simulink model "ACC"  (R2022b)
settings: Solver=FixedStepDiscrete  StartTime=0.0  StopTime=10.0  FixedStep=0.01  RelTol=1e-3
libraries: simulink x1
settings Model: DataDictionary=Adaptive_Cruise_Control.sldd  Creator=MAAM  LastModifiedBy=MAAM
settings OptimizationCC: DefaultParameterBehavior=Inlined  UseDivisionForNetSlopeComputation=on  GainParamInheritBuiltInType=on  UseFloatMulNetSlope=on  InlineInvariantSignals=on  PassReuseOutputArgsAs=Individual arguments  ZeroExternalMemoryAtStartup=off  ZeroInternalMemoryAtStartup=off  NoFixptDivByZeroProtection=on  EfficientFloat2IntCast=on  LifeSpan=1  OptimizeBlockOrder=speed  DifferentSizesBufferReuse=on  EfficientTunableParamExpr=on
settings DebuggingCC: ParameterTunabilityLossMsg=error
settings HardwareCC: ProdBitPerPointer=32  ProdBitPerSizeT=32  ProdBitPerPtrDiffT=32  ProdLargestAtomicInteger=Long  ProdLargestAtomicFloat=Double  ProdWordSize=32  ProdLongLongMode=on  ProdHWDeviceType=ARM Compatible->ARM Cortex-M
settings SFSimCC: MATLABDynamicMemAlloc=off
settings RTWCC: Description=Embedded Coder  SystemTargetFile=ert.tlc  GenCodeOnly=on  TemplateMakefile=ert_default_tmf
settings CodeAppCC: ForceParamTrailComments=on  IgnoreCustomStorageClasses=off  OperatorAnnotations=on  SimulinkDataObjDesc=on  SFDataObjDesc=on  CustomSymbolStrGlobalVar=rt$N$M  CustomSymbolStrType=$N$M  CustomSymbolStrFcn=$N$M$F  CustomSymbolStrMacro=$N$M  InsertBlockDesc=on
settings ERTTargetCC: TargetLangStandard=C99 (ISO)  GenerateSampleERTMain=on  IncludeMdlTerminateFcn=off  CombineSignalStateStructs=on  SupportAbsoluteTime=off  SupportComplex=off  SupportNonInlinedSFcns=on  InlinedParameterPlacement=NonHierarchical  ERTCustomFileTemplate=example_file_process.tlc  ERTFilePackagingFormat=CompactWithDataFile

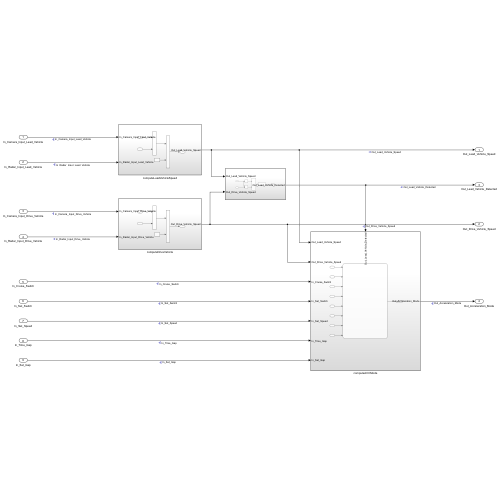
[thumbnail: Simulink's stored preview of the top-level diagram]
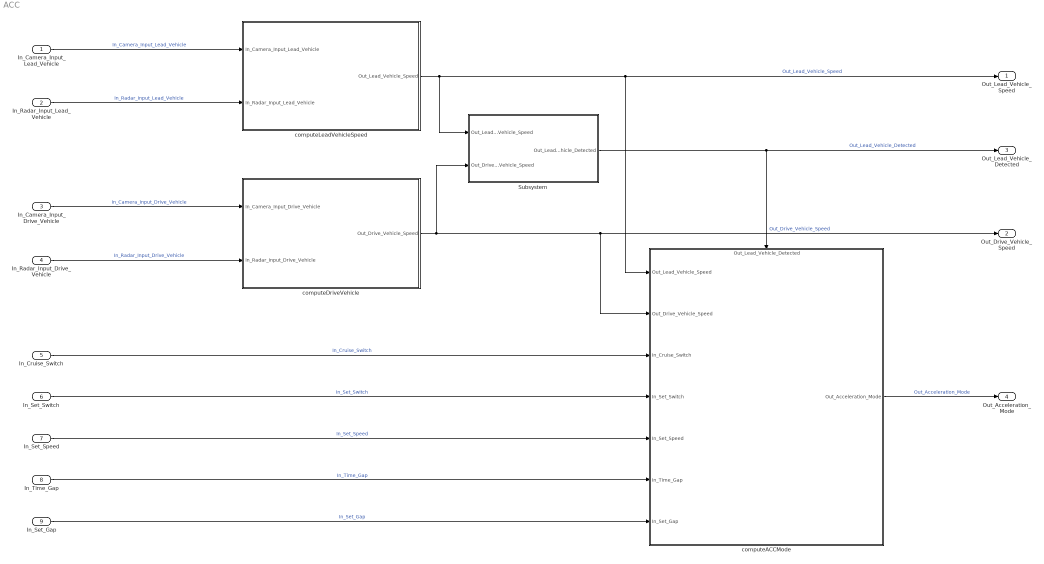
== system ACC ==
  In_Camera_Input_Lead_Vehicle : Inport  OutDataTypeStr=uint8
  In_Radar_Input_Lead_Vehicle : Inport  Port=2  OutDataTypeStr=uint8
  In_Camera_Input_Drive_Vehicle : Inport  Port=3  OutDataTypeStr=uint8
  In_Radar_Input_Drive_Vehicle : Inport  Port=4  OutDataTypeStr=uint8
  In_Cruise_Switch : Inport  Port=5  OutDataTypeStr=boolean
  In_Set_Switch : Inport  Port=6  OutDataTypeStr=boolean
  In_Set_Speed : Inport  Port=7  OutDataTypeStr=uint8
  In_Time_Gap : Inport  Port=8  OutDataTypeStr=uint8
  In_Set_Gap : Inport  Port=9  OutDataTypeStr=uint8
  Subsystem : Subsystem
  computeACCMode : Subsystem
      settings: PortSchema="{\"entries\":[{\"content\":{\"sides\":[{\"content\":{\"connectorIds\":[\"In1\",\"In2\",\"In3\",\"In4\",\"In5\",\"In6\",\"In7\"]},\"type\":\"ConnectorPlacement.EquallySpacedRectSide\",\"uuid\":\"34e4527d-3073-4040-9a65-5b2192b0ac7a\"},{\"content\":{\"connectorIds\":[\"Out1\"],\"side\":\"RIGHT\"},\"type\":\"ConnectorPlacement.EquallySpacedRectSide\",\"uuid\":\"d28eb757-50b9-4815-93ce-88b039d8e03c\"},{\"content\":{\"connectorIds\":[\"In8\"],\"side\":\"TOP\"},\"type\":\"ConnectorPlacement.EquallySpacedRectSide\",\"uuid\":\"9f5a8a03-fc12-423c-b68a-6a82dedc6e29\"}]},\"type\":\"ConnectorPlacement.EquallySpacedConnector\",\"uuid\":\"64ab1c3b-0e5f-41ed-aa52-f96656837c78\"}],\"packageUris\":[\"http://schema.mathworks.com/mf0/Connector/R2020b\"],\"version\":\"1.0\"}"
  computeDriveVehicle : Subsystem
  computeLeadVehicleSpeed : Subsystem
  Out_Lead_Vehicle_Speed : Outport  OutDataTypeStr=uint8
  Out_Drive_Vehicle_Speed : Outport  Port=2  OutDataTypeStr=uint8
  Out_Lead_Vehicle_Detected : Outport  Port=3  OutDataTypeStr=uint8
  Out_Acceleration_Mode : Outport  Port=4  OutDataTypeStr=uint8
  wires:
  computeLeadVehicleSpeed/1(Out_Lead_Vehicle_Speed) -> Subsystem/1(Out_Lead_Vehicle_Speed), Out_Lead_Vehicle_Speed/1, computeACCMode/1(Out_Lead_Vehicle_Speed)  "Out_Lead_Vehicle_Speed"
  In_Camera_Input_Lead_Vehicle/1 -> computeLeadVehicleSpeed/1(In_Camera_Input_Lead_Vehicle)  "In_Camera_Input_Lead_Vehicle"
  In_Radar_Input_Lead_Vehicle/1 -> computeLeadVehicleSpeed/2(In_Radar_Input_Lead_Vehicle)  "In_Radar_Input_Lead_Vehicle"
  computeDriveVehicle/1(Out_Drive_Vehicle_Speed) -> Out_Drive_Vehicle_Speed/1, computeACCMode/2(Out_Drive_Vehicle_Speed), Subsystem/2(Out_Drive_Vehicle_Speed)  "Out_Drive_Vehicle_Speed"
  computeACCMode/1(Out_Acceleration_Mode) -> Out_Acceleration_Mode/1  "Out_Acceleration_Mode"
  In_Cruise_Switch/1 -> computeACCMode/3(In_Cruise_Switch)  "In_Cruise_Switch"
  In_Set_Switch/1 -> computeACCMode/4(In_Set_Switch)  "In_Set_Switch"
  In_Set_Speed/1 -> computeACCMode/5(In_Set_Speed)  "In_Set_Speed"
  In_Time_Gap/1 -> computeACCMode/6(In_Time_Gap)  "In_Time_Gap"
  In_Set_Gap/1 -> computeACCMode/7(In_Set_Gap)  "In_Set_Gap"
  In_Radar_Input_Drive_Vehicle/1 -> computeDriveVehicle/2(In_Radar_Input_Drive_Vehicle)  "In_Radar_Input_Drive_Vehicle"
  In_Camera_Input_Drive_Vehicle/1 -> computeDriveVehicle/1(In_Camera_Input_Drive_Vehicle)  "In_Camera_Input_Drive_Vehicle"
  Subsystem/1(Out_Lead_Vehicle_Detected) -> Out_Lead_Vehicle_Detected/1, computeACCMode/8(Out_Lead_Vehicle_Detected)  "Out_Lead_Vehicle_Detected"

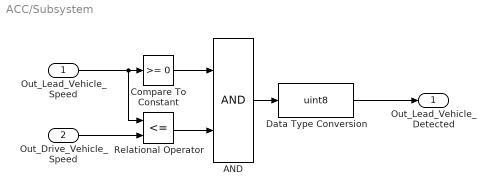
== system ACC/Subsystem ==
  Out_Lead_Vehicle_Speed : Inport  OutDataTypeStr=uint8
  Out_Drive_Vehicle_Speed : Inport  Port=2  OutDataTypeStr=uint8
  AND : Logic  AllPortsSameDT=off  OutDataTypeStr=boolean
  Compare To Constant : simulink/Logic and Bit Operations/Compare To Constant  relop=>=  const=0  OutDataTypeStr=boolean
  Data Type Conversion : DataTypeConversion  OutDataTypeStr=uint8  SaturateOnIntegerOverflow=off  RndMeth=Floor
  Relational Operator : RelationalOperator  Operator=<=  OutDataTypeStr=boolean  RndMeth=Simplest  InputSameDT=off
  Out_Lead_Vehicle_Detected : Outport  OutDataTypeStr=uint8
  wires:
  Out_Lead_Vehicle_Speed/1 -> Relational Operator/1, Compare To Constant/1
  Out_Drive_Vehicle_Speed/1 -> Relational Operator/2
  Compare To Constant/1 -> AND/1
  Relational Operator/1 -> AND/2
  AND/1 -> Data Type Conversion/1
  Data Type Conversion/1 -> Out_Lead_Vehicle_Detected/1

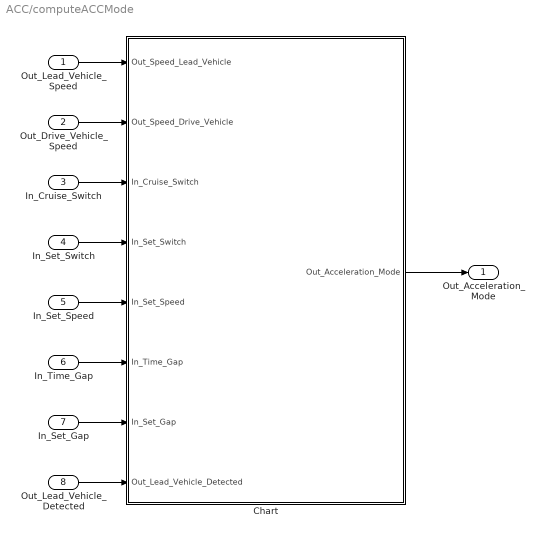
== system ACC/computeACCMode ==
  Out_Lead_Vehicle_Speed : Inport
  Out_Drive_Vehicle_Speed : Inport  Port=2
  In_Cruise_Switch : Inport  Port=3  OutDataTypeStr=boolean
  In_Set_Switch : Inport  Port=4  OutDataTypeStr=boolean
  In_Set_Speed : Inport  Port=5  OutDataTypeStr=uint8
  In_Time_Gap : Inport  Port=6  OutDataTypeStr=uint8
  In_Set_Gap : Inport  Port=7  OutDataTypeStr=uint8
  Out_Lead_Vehicle_Detected : Inport  Port=8  OutDataTypeStr=uint8
  Chart : Stateflow chart  TreatAsAtomicUnit=on
      settings: PortSchema="{\"entries\":[{\"content\":{\"sides\":[{\"content\":{\"connectorIds\":[\"In2\",\"In3\",\"In4\",\"In5\",\"In6\",\"In7\",\"In8\",\"In1\"]},\"type\":\"ConnectorPlacement.EquallySpacedRectSide\",\"uuid\":\"34e4527d-3073-4040-9a65-5b2192b0ac7a\"},{\"content\":{\"connectorIds\":[\"Out1\"],\"side\":\"RIGHT\"},\"type\":\"ConnectorPlacement.EquallySpacedRectSide\",\"uuid\":\"d28eb757-50b9-4815-93ce-88b039d8e03c\"},{\"content\":{\"connectorIds\":[],\"side\":\"TOP\"},\"type\":\"ConnectorPlacement.EquallySpacedRectSide\",\"uuid\":\"9f5a8a03-fc12-423c-b68a-6a82dedc6e29\"},{\"content\":{\"connectorIds\":[],\"side\":\"BOTTOM\"},\"type\":\"ConnectorPlacement.EquallySpacedRectSide\",\"uuid\":\"fb5576b8-ca7b-42c5-8f28-21c14c714186\"}]},\"type\":\"ConnectorPlacement.EquallySpacedConnector\",\"uuid\":\"64ab1c3b-0e5f-41ed-aa52-f96656837c78\"}],\"packageUris\":[\"http://schema.mathworks.com/mf0/Connector/R2020b\"],\"version\":\"1.0\"}"
  Out_Acceleration_Mode : Outport  OutDataTypeStr=uint8
  wires:
  In_Set_Gap/1 -> Chart/8(In_Set_Gap)
  In_Time_Gap/1 -> Chart/7(In_Time_Gap)
  In_Set_Speed/1 -> Chart/6(In_Set_Speed)
  In_Set_Switch/1 -> Chart/5(In_Set_Switch)
  In_Cruise_Switch/1 -> Chart/4(In_Cruise_Switch)
  Chart/1(Out_Acceleration_Mode) -> Out_Acceleration_Mode/1
  Out_Lead_Vehicle_Speed/1 -> Chart/2(Out_Speed_Lead_Vehicle)
  Out_Drive_Vehicle_Speed/1 -> Chart/3(Out_Speed_Drive_Vehicle)
  Out_Lead_Vehicle_Detected/1 -> Chart/1(Out_Lead_Vehicle_Detected)

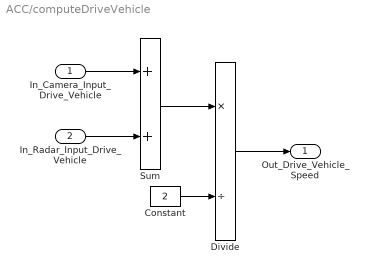
== system ACC/computeDriveVehicle ==
  In_Camera_Input_Drive_Vehicle : Inport  OutDataTypeStr=uint8
  In_Radar_Input_Drive_Vehicle : Inport  Port=2  OutDataTypeStr=uint8
  Constant : Constant  Value=2
  Divide : Product  Inputs=*/  OutDataTypeStr=uint8  RndMeth=Round
  Sum : Sum
  Out_Drive_Vehicle_Speed : Outport  OutDataTypeStr=uint8
  wires:
  Divide/1 -> Out_Drive_Vehicle_Speed/1
  In_Radar_Input_Drive_Vehicle/1 -> Sum/2
  In_Camera_Input_Drive_Vehicle/1 -> Sum/1
  Sum/1 -> Divide/1
  Constant/1 -> Divide/2

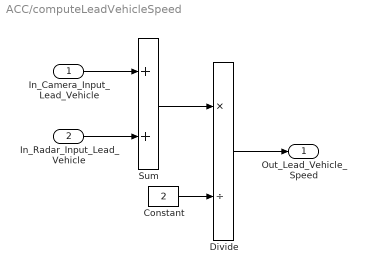
== system ACC/computeLeadVehicleSpeed ==
  In_Camera_Input_Lead_Vehicle : Inport  OutDataTypeStr=uint8
  In_Radar_Input_Lead_Vehicle : Inport  Port=2  OutDataTypeStr=uint8
  Constant : Constant  Value=2
  Divide : Product  Inputs=*/  OutDataTypeStr=uint8  RndMeth=Round
  Sum : Sum
  Out_Lead_Vehicle_Speed : Outport  OutDataTypeStr=uint8
  wires:
  In_Camera_Input_Lead_Vehicle/1 -> Sum/1
  In_Radar_Input_Lead_Vehicle/1 -> Sum/2
  Sum/1 -> Divide/1
  Divide/1 -> Out_Lead_Vehicle_Speed/1
  Constant/1 -> Divide/2

== stateflow chart ACC/computeACCMode/Chart ==
  state ACC_OFF_MODE
    en:
    Out_Acceleration_Mode = uint8(0);
  state ACC_STANDBY_MODE
    en:
    Out_Acceleration_Mode = uint8(1);
  state ACC_ON_MODE
    state Lead_Vehicle_Detected_Follow
      en:
      Out_Acceleration_Mode = uint8(2);
    state Lead_Vehicle_Not_Detected
      en:
      Out_Acceleration_Mode = uint8(1);
    state Lead_Vehicle_Speed_Less_Than_Set_Speed
      en:
      Out_Acceleration_Mode = uint8(4);
    state Lead_Vehicle_Detected_Resume
      en:
      Out_Acceleration_Mode = uint8(3);
    state Lead_Vehicle_Speed_Equal_Set_Speed
      en:
      Out_Acceleration_Mode = uint8(5);
    state Lead_Vehicle_Not_Detected_Resume
      en:
      Out_Acceleration_Mode = uint8(1);
    (default) -> Lead_Vehicle_Detected_Follow
    Lead_Vehicle_Not_Detected -> Lead_Vehicle_Detected_Follow [order 1] : [( Out_Lead_Vehicle_Detected == 1 ) && ...
        |  ( Out_Speed_Drive_Vehicle == In_Set_Speed ) && ...
        |  ( Out_Speed_Lead_Vehicle >= In_Set_Speed ) && ...
        |  ( In_Time_Gap >= In_Set_Gap )]
    Lead_Vehicle_Detected_Follow -> Lead_Vehicle_Not_Detected [order 1] : [Out_Lead_Vehicle_Detected == 0]
    Lead_Vehicle_Speed_Less_Than_Set_Speed -> Lead_Vehicle_Not_Detected [order 1] : [( Out_Lead_Vehicle_Detected == 0 ) && ...
        | ( Out_Speed_Drive_Vehicle == In_Set_Speed )]
    Lead_Vehicle_Not_Detected -> Lead_Vehicle_Speed_Less_Than_Set_Speed [order 2] : [( Out_Lead_Vehicle_Detected == 1 ) && ...
        |  ( Out_Speed_Lead_Vehicle < In_Set_Speed ) || ...
        |  ( In_Time_Gap < In_Set_Gap )]
    Lead_Vehicle_Detected_Follow -> Lead_Vehicle_Speed_Less_Than_Set_Speed [order 2] : [( Out_Lead_Vehicle_Detected == 1 ) && ...
        |  ( Out_Speed_Lead_Vehicle < In_Set_Speed ) || ...
        |  ( In_Time_Gap < In_Set_Gap )]
    Lead_Vehicle_Detected_Resume -> Lead_Vehicle_Detected_Follow [order 1] : [( Out_Speed_Drive_Vehicle == In_Set_Speed ) && ...
        |  ( Out_Speed_Lead_Vehicle >= In_Set_Speed ) && ...
        |  ( In_Time_Gap >= In_Set_Gap )]
    Lead_Vehicle_Speed_Equal_Set_Speed -> Lead_Vehicle_Speed_Less_Than_Set_Speed [order 3] : [( Out_Speed_Lead_Vehicle < In_Set_Speed ) && ...
        |  ( Out_Speed_Lead_Vehicle < Out_Speed_Drive_Vehicle ) || ...
        |  ( In_Time_Gap == 0.75 * In_Set_Gap )]
    Lead_Vehicle_Speed_Less_Than_Set_Speed -> Lead_Vehicle_Speed_Equal_Set_Speed [order 2] : [( Out_Speed_Lead_Vehicle * 1.25 >= Out_Speed_Drive_Vehicle ) && ...
        |  ( Out_Speed_Lead_Vehicle * 0.75 <= Out_Speed_Drive_Vehicle ) && ...
        |  ( Out_Speed_Drive_Vehicle < In_Set_Speed ) && ( In_Time_Gap <= 1.25 * In_Set_Gap ) && ...
        |  ( In_Time_Gap >= 0.75 * In_Set_Gap )]
    Lead_Vehicle_Speed_Equal_Set_Speed -> Lead_Vehicle_Detected_Resume [order 2] : [( Out_Speed_Drive_Vehicle < In_Set_Speed ) && ...
        | ( Out_Speed_Lead_Vehicle > Out_Speed_Drive_Vehicle ) || ...
        | ( In_Time_Gap >= In_Set_Gap )]
    Lead_Vehicle_Detected_Resume -> Lead_Vehicle_Speed_Equal_Set_Speed [order 3] : [( Out_Speed_Drive_Vehicle < In_Set_Speed ) && ...
        |  ( Out_Speed_Lead_Vehicle > Out_Speed_Drive_Vehicle ) && ...
        |  ( In_Time_Gap >= In_Set_Gap )]
    Lead_Vehicle_Speed_Equal_Set_Speed -> Lead_Vehicle_Not_Detected_Resume [order 1] : [( Out_Lead_Vehicle_Detected == 0 ) || ...
        |  ( Out_Speed_Drive_Vehicle <= In_Set_Speed )]
    Lead_Vehicle_Detected_Resume -> Lead_Vehicle_Not_Detected_Resume [order 2] : [Out_Lead_Vehicle_Detected == 0]
  (default) -> ACC_OFF_MODE
  ACC_STANDBY_MODE -> ACC_OFF_MODE [order 1] : [In_Set_Switch == 0]
  ACC_OFF_MODE -> ACC_STANDBY_MODE : [In_Cruise_Switch == 1]
  ACC_ON_MODE -> ACC_OFF_MODE : [In_Cruise_Switch == 0]
  ACC_STANDBY_MODE -> ACC_ON_MODE [order 2] : [In_Set_Switch == 1]
  data: Out_Lead_Vehicle_Detected input; Out_Speed_Lead_Vehicle input; Out_Speed_Drive_Vehicle input; In_Cruise_Switch input; In_Set_Switch input; In_Set_Speed input; In_Time_Gap input; In_Set_Gap input; Out_Acceleration_Mode output
